simulink model "Project"  (R2020a)
settings: Solver=VariableStepAuto  StartTime=0.0  StopTime=20  RelTol=1e-3
libraries: arduinolib x13, simulink x1
settings Model: Creator=hend_aafia  LastModifiedBy=hend_aafia

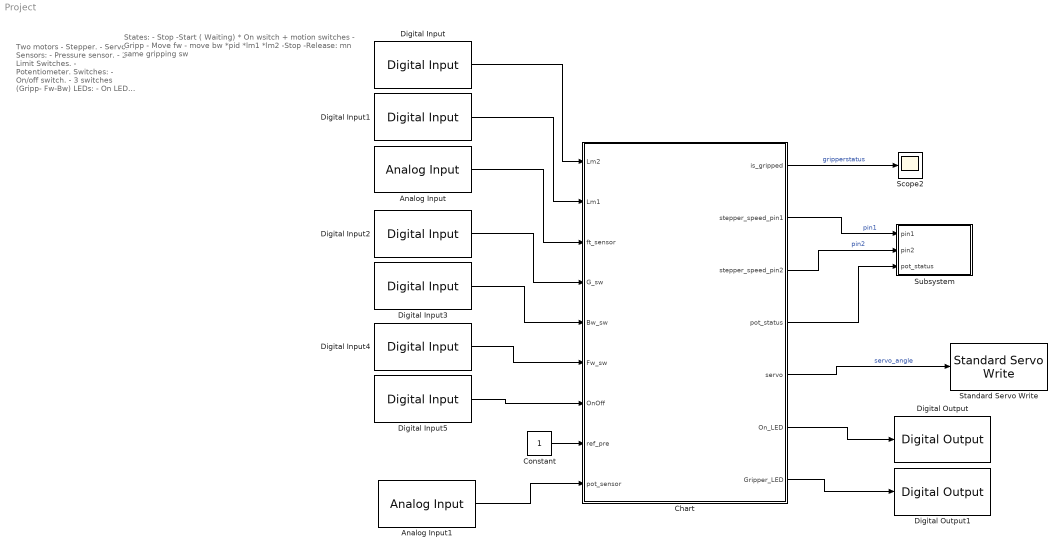
== system Project ==
  note: Two motors
      | - Stepper.
      | - Servo.
      |
      | Sensors:
      | - Pressure sensor.
      | - 2 Limit Switches.
      | - Potentiometer.
      |
      | Switches:
      | - On/off switch.
      | - 3 switches (Gripp- Fw-Bw)
      |
      | LEDs:
      | - On LED
      | - Gripper LED
      |
      | - Gripper LED
      | - Fw LED
      | - Bw LED
  note: States:
      | - Stop
      | -Start ( Waiting)
      |
      | * On wsitch + motion switches
      |
      | - Gripp - Move fw - move bw
      |
      | *pid *lm1 *lm2
      |
      | -Stop
      | -Release:
      | mn same gripping sw
  Analog Input : arduinolib/Analog Input  pinNumber=0  ReadResultsOnly=off  ConversionTriggerSource=Software  ExternalTriggerType=uint32( 0 )  OutputDataType=uint16  EnableConversionCompleteNotify=off  EnableOuputStatus=off  SampleTime=-1  blockPlatform=arduino
  Analog Input1 : arduinolib/Analog Input  pinNumber=0  ReadResultsOnly=off  ConversionTriggerSource=Software  ExternalTriggerType=uint32( 0 )  OutputDataType=uint16  EnableConversionCompleteNotify=off  EnableOuputStatus=off  SampleTime=-1  blockPlatform=arduino
  Chart : Stateflow chart  TreatAsAtomicUnit=on
  Constant : Constant
  Digital Input : arduinolib/Digital Input  pinNumber=4  Direction=input  SampleTime=0.1  blockPlatform=arduino
  Digital Input1 : arduinolib/Digital Input  pinNumber=5  Direction=input  SampleTime=0.1  blockPlatform=arduino
  Digital Input2 : arduinolib/Digital Input  pinNumber=8  Direction=input  SampleTime=0.1  blockPlatform=arduino
  Digital Input3 : arduinolib/Digital Input  pinNumber=6  Direction=input  SampleTime=0.1  blockPlatform=arduino
  Digital Input4 : arduinolib/Digital Input  pinNumber=7  Direction=input  SampleTime=0.1  blockPlatform=arduino
  Digital Input5 : arduinolib/Digital Input  pinNumber=10  Direction=input  SampleTime=0.1  blockPlatform=arduino
  Digital Output : arduinolib/Digital Output  pinNumber=9  Direction=output  blockPlatform=arduino
  Digital Output1 : arduinolib/Digital Output  pinNumber=9  Direction=output  blockPlatform=arduino
  Scope2 : Scope
  Standard Servo Write : arduinolib/Standard Servo Write  pinNumber=9  ServoIndex=0  blockPlatform=ARDUINO
  Subsystem : Subsystem
  wires:
  Chart/5(servo) -> Standard Servo Write/1  "servo_angle"
  Digital Input/1 -> Chart/1(Lm2)
  Digital Input3/1 -> Chart/5(Bw_sw)
  Digital Input5/1 -> Chart/7(OnOff)
  Chart/1(is_gripped) -> Scope2/1  "gripperstatus"
  Chart/6(On_LED) -> Digital Output/1
  Chart/7(Gripper_LED) -> Digital Output1/1
  Constant/1 -> Chart/8(ref_pre)
  Digital Input1/1 -> Chart/2(Lm1)
  Digital Input2/1 -> Chart/4(G_sw)
  Digital Input4/1 -> Chart/6(Fw_sw)
  Analog Input/1 -> Chart/3(ft_sensor)
  Analog Input1/1 -> Chart/9(pot_sensor)
  Chart/4(pot_status) -> Subsystem/3(pot_status)
  Chart/2(stepper_speed_pin1) -> Subsystem/1(pin1)  "pin1"
  Chart/3(stepper_speed_pin2) -> Subsystem/2(pin2)  "pin2"

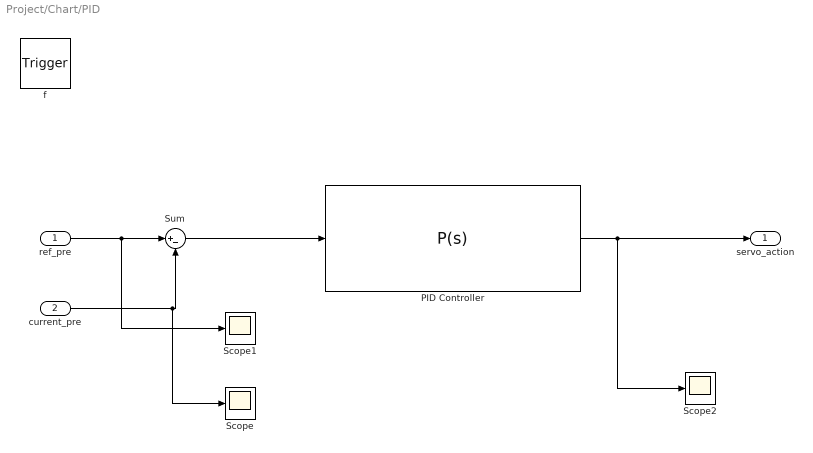
== system Project/Chart/PID ==
  ref_pre : Inport  OutMin=-1000  OutMax=1000  OutDataTypeStr=double  Unit=N/(m^2)  PortDimensions=1
  current_pre : Inport  Port=2  OutDataTypeStr=double  Unit=N/(m^2)  PortDimensions=1
  f : TriggerPort  TriggerType=function-call  VariantControl=(inherit)
      settings: CopyFcn=Stateflow.SLINSF.SimulinkMan.removeBlockPreDeleteFcn  PreDeleteFcn=Stateflow.SLINSF.SimulinkMan.unsafePredeleteFcn
  PID Controller : simulink/Continuous/PID Controller  Controller=P  Form=Parallel  TimeDomain=Continuous-time  UseExternalTs=off  SampleTime=-1  IntegratorMethod=Forward Euler  FilterMethod=Forward Euler  ControllerParametersSource=internal  P=1  I=1  D=0  UseFilter=on  N=100  TunerSelectOption=Transfer Function Based (PID Tuner App)  InitialConditionSource=internal  InitialConditionForIntegrator=0  InitialConditionForFilter=0  DifferentiatorICPrevScaledInput=0  ExternalReset=none  TrackingMode=off  Kt=1  LimitOutput=off  UpperSaturationLimit=inf  LowerSaturationLimit=-inf  LinearizeAsGain=on  AntiWindupMode=none  Kb=1  POutMin=[]  POutMax=[]  IOutMin=[]  IOutMax=[]  DOutMin=[]  DOutMax=[]  NOutMin=[]  NOutMax=[]  SumOutMin=[]  SumOutMax=[]  SaturationOutMin=[]  SaturationOutMax=[]  PParamMin=[]  PParamMax=[]  IParamMin=[]  IParamMax=[]  DParamMin=[]  DParamMax=[]  NParamMin=[]  NParamMax=[]  KbParamMin=[]  KbParamMax=[]  KtParamMin=[]  KtParamMax=[]  KbOutMin=[]  KbOutMax=[]  KtOutMin=[]  KtOutMax=[]  IntegratorOutMin=[]  IntegratorOutMax=[]  FilterOutMin=[]  FilterOutMax=[]  SumI1OutMin=[]  SumI1OutMax=[]  SumI2OutMin=[]  SumI2OutMax=[]  SumI3OutMin=[]  SumI3OutMax=[]  SumI4OutMin=[]  SumI4OutMax=[]  SumDOutMin=[]  SumDOutMax=[]  DifferentiatorOutMin=[]  DifferentiatorOutMax=[]  FilterDiffOutCoefMin=[]  FilterDiffOutCoefMax=[]  ReciprocalOutMin=[]  ReciprocalOutMax=[]  SumDenOutMin=[]  SumDenOutMax=[]  SumNumOutMin=[]  SumNumOutMax=[]  DivideOutMin=[]  DivideOutMax=[]  UdiffTsProdOutMin=[]  UdiffTsProdOutMax=[]  NTsProdOutMin=[]  NTsProdOutMax=[]  UintegralTsProdOutMin=[]  UintegralTsProdOutMax=[]  UngainTsProdOutMin=[]  UngainTsProdOutMax=[]  IntegratorContinuousStateAttributes=''  IntegratorStateMustResolveToSignalObject=off  IntegratorRTWStateStorageClass=Auto  FilterContinuousStateAttributes=''  FilterStateMustResolveToSignalObject=off  FilterRTWStateStorageClass=Auto  ParallelPVariant=InternalParameters  IdealPVariant=Disabled  IVariant=Disabled  DVariant=Disabled  IntegratorVariant=Disabled  SatVariant=Disabled  AWVariant=Disabled  PCopyVariant=Disabled  TRVariant=Disabled  FdbkBlocksVariant=Forward  IdealPFdbkVariant=Disabled  SatFdbkVariant=Disabled  DerivativeFilterVariant=Disabled  NVariant=Disabled  NCopyVariant=Disabled_SignalSpec  FilterICVariant=Disabled  IntegratorICVariant=Disabled  ExternalResetVariant=Disabled  TRSumVariant=Passthrough  SumFdbkVariant=Disabled  SumVariant=Passthrough_P  TsampFilterVariant=InternalTs  TsampNgainVariant=Passthrough  TsampIntegralVariant=Disabled_SignalSpec
  Scope : Scope
  Scope1 : Scope
  Scope2 : Scope
  Sum : Sum  Inputs=|+-
  servo_action : Outport
  wires:
  ref_pre/1 -> Scope1/1, Sum/1
  Sum/1 -> PID Controller/1
  PID Controller/1 -> Scope2/1, servo_action/1
  current_pre/1 -> Scope/1, Sum/2

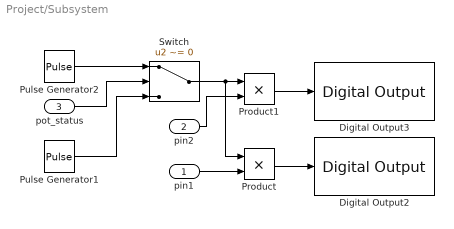
== system Project/Subsystem ==
  pin1 : Inport
  pin2 : Inport  Port=2
  pot_status : Inport  Port=3
  Digital Output2 : arduinolib/Digital Output  pinNumber=3  Direction=output  blockPlatform=arduino
  Digital Output3 : arduinolib/Digital Output  pinNumber=2  Direction=output  blockPlatform=arduino
  Product : Product
  Product1 : Product
  Pulse Generator1 : DiscretePulseGenerator  PulseType=Time based  Period=1  PulseWidth=50
  Pulse Generator2 : DiscretePulseGenerator  PulseType=Time based  Period=1  PulseWidth=50
  Switch : Switch  Criteria=u2 ~= 0
  wires:
  Pulse Generator1/1 -> Switch/3
  Switch/1 -> Product/1, Product1/1
  Product1/1 -> Digital Output3/1
  pin2/1 -> Product1/2
  pin1/1 -> Product/2
  Pulse Generator2/1 -> Switch/1
  Product/1 -> Digital Output2/1
  pot_status/1 -> Switch/2

== stateflow chart Project/Chart ==
  state Stop
    en:
    is_gripped = 0;
    On_LED =0;
    for pos = [70:1:160]
    servo = pos;
    end
  state servo_action = PID(ref_pre,current_pre) [function]
  state Gripper
    en:
    is_gripped = 1;
    Gripper_LED = 1;
    during:
    servo = PID(ref_pre,ft_sensor);
    if (ft_sensor > ref_pre || ft_sensor == ref_pre || abs(ref_pre - ft_sensor) <0.1)
    PID_done = 1;
    end
  state FW
    during:
    stepper_speed_pin1 = 1;
    stepper_speed_pin2 = 0;
  state Start
    en:
    PID_done =0;
    stepper_speed = 0;
    On_LED =1;
    Gripper_LED = 0;
    if pot_sensor > 100
    pot_status = 0;
    else
    pot_status =1;
    end
  state Release
    en:
    is_gripped =0;
    during:
    for pos = [70:1:160]
    servo = pos;
    end
  state BW
    during:
    stepper_speed_pin1 = 0;
    stepper_speed_pin2 = 1;
  (default) -> Stop
  Release -> Stop [order 1] : [OnOff == 0]
  Gripper -> Stop [order 1] : [OnOff == 0]
  BW -> Stop [order 1] : [OnOff == 0]
  FW -> Stop [order 1] : [OnOff ==0]
  Start -> Stop [order 1] : [OnOff==0]
  Stop -> Start : [OnOff==1]
  Start -> FW [order 2] : [Fw_sw ==1 && Lm1 == 0]
  Start -> Gripper [order 4] : [(G_sw == 1) && (is_gripped == 0)]
  Gripper -> Start [order 2] : [PID_done == 1]
  FW -> Start [order 2] : [Lm1 == 1]
  Release -> Start [order 2] : [ft_sensor==0]
  Start -> Release [order 5] : [(G_sw == 1) && (is_gripped == 1)]
  BW -> Start [order 2] : [Lm2==1]
  Start -> BW [order 3] : [Bw_sw == 1]
  data: ref_pre function_input double size=1; current_pre function_input double size=1; servo_action function_output; Lm2 input; Lm1 input; ft_sensor input; is_gripped output; G_sw input; Bw_sw input; Fw_sw input; OnOff input; stepper_speed_pin1 output; stepper_speed_pin2 output; pot_status output; servo output; PID_done local; On_LED output; Gripper_LED output; ref_pre input; pos local; pot_sensor input
